simulink model "Energy_Cost"  (Simulink 8.8)
settings: Solver=ode23t  StartTime=0.0  StopTime=24  RelTol=1e-3  EnableMultiTasking=on
model workspace: external: MAT-File (data not in the file)
libraries: simulink x4
(part 2 of 5)

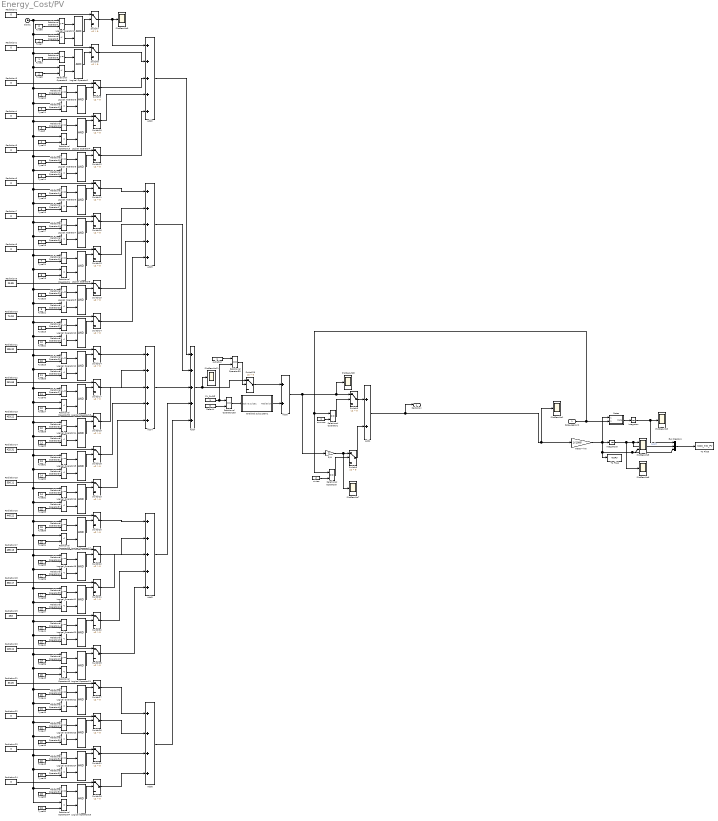
== system Energy_Cost/PV ==
  Rate_season2 : Inport
  Add1 : Sum
  Add{2..5,7} (5 alike) : Sum  Inputs=+++++
  Add6 : Sum  Inputs=++++
  Add8 : Sum
  Bus Creator4 : BusCreator  Inputs=3
  Clock1 : Clock
  Default : Constant  Value=0
  Enabled Subsystem1 : Subsystem  TreatAsAtomicUnit=on
  Integrator : Integrator
  Integrator3 : Integrator
  Logical Operator{1..18,20..25} (24 alike) : Logic  AllPortsSameDT=off  OutDataTypeStr=boolean
  PV_OnOff : Constant
  PlotResults{1,3,6..9,11} (7 alike) : Scope
  PlotResults5 : Scope  NumInputPorts=2
  Radiation{1..8,22..24} (11 alike) : Constant  Value=0
  Radiation10 : Constant  Value=74.18
  Radiation11 : Constant  Value=195.32
  Radiation12 : Constant  Value=281.63
  Radiation13 : Constant  Value=453.22
  Radiation14 : Constant  Value=425.31
  Radiation15 : Constant  Value=556.11
  Radiation16 : Constant  Value=445.22
  Radiation17 : Constant  Value=485.13
  Radiation18 : Constant  Value=360.17
  Radiation19 : Constant  Value=253
  Radiation20 : Constant  Value=126.11
  Radiation21 : Constant  Value=33.25
  Radiation9 : Constant  Value=25.85
  Rates : Subsystem
  Relational Operator{1,5,55,103} (4 alike) : RelationalOperator  Operator===  RndMeth=Nearest  InputSameDT=on
  Relational Operator{6..7,10..11,14..15,18..19,22..23,27..28,31..32,35..36,39..40,43..44,47..48,51..52} (24 alike) : RelationalOperator  RndMeth=Nearest  InputSameDT=on
  Relational Operator{8..9,12..13,16..17,20..21,25..26,29..30,33..34,37..38,41..42,45..46,49..50,53..54} (24 alike) : RelationalOperator  Operator=<  RndMeth=Nearest  InputSameDT=on
  S\W : Gain  Gain=.5  SaturateOnIntegerOverflow=on  OutDataTypeStr=Inherit: Same as input  ParamDataTypeStr=Inherit: Same as input
  Switch{5..29,31..32} (27 alike) : Switch  Criteria=u2 > Threshold
  To File1 : ToFile  Filename=TinPV  MatrixName=TinPV
  To File5 : ToFile  Filename=Cost_KW_PV  MatrixName=Cost_KW_PV
  Type10 : Constant  Value=2
  Type11 : Constant  Value=3
  Type12 : Constant  Value=4
  Type13 : Constant  Value=4
  Type14 : Constant  Value=5
  Type15 : Constant  Value=6
  Type16 : Constant  Value=5
  Type17 : Constant  Value=6
  Type18 : Constant  Value=7
  Type19 : Constant  Value=8
  Type2 : Constant
  Type20 : Constant  Value=8
  Type21 : Constant  Value=9
  Type22 : Constant  Value=10
  Type23 : Constant  Value=9
  Type24 : Constant  Value=7
  Type25 : Constant  Value=10
  Type26 : Constant  Value=11
  Type27 : Constant  Value=12
  Type28 : Constant  Value=12
  Type29 : Constant  Value=13
  Type30 : Constant  Value=14
  Type31 : Constant  Value=13
  Type32 : Constant  Value=14
  Type33 : Constant  Value=15
  Type34 : Constant  Value=16
  Type35 : Constant  Value=16
  Type36 : Constant  Value=17
  Type37 : Constant  Value=18
  Type38 : Constant  Value=17
  Type39 : Constant  Value=15
  Type40 : Constant  Value=11
  Type41 : Constant  Value=18
  Type42 : Constant  Value=19
  Type43 : Constant  Value=20
  Type44 : Constant  Value=20
  Type45 : Constant  Value=21
  Type46 : Constant  Value=22
  Type47 : Constant  Value=21
  Type48 : Constant  Value=22
  Type49 : Constant  Value=23
  Type50 : Constant  Value=24
  Type55 : Constant  Value=23
  Type56 : Constant  Value=19
  Type6 : Constant  Value=0
  Type7 : Constant
  Type8 : Constant  Value=2
  Type9 : Constant  Value=3
  Watts-->kW : Gain  Gain=1/(1000)  SaturateOnIntegerOverflow=on  OutDataTypeStr=Inherit: Same as input  ParamDataTypeStr=Inherit: Same as input
  radiation : Constant
  summer : Constant
  winter : Constant  Value=2
  Radiation : Outport
  wires:
  Add1/1 -> PlotResults1/1, Watts-->kW/1, Radiation/1
  Integrator3/1 -> PlotResults5/1, Bus Creator4/2, PlotResults6/1  "kw-hr"
  Watts-->kW/1 -> Integrator3/1, Rates/1(Powe_cons), To File1/1, Bus Creator4/3, PlotResults5/2
  Rates/1(Rate) -> Integrator/1
  Integrator/1 -> PlotResults3/1, Bus Creator4/1
  Rate_season2/1 -> Rates/2(Rate_season2), Relational Operator1/1, Relational Operator5/1
  Relational Operator1/1 -> Switch5/2
  summer/1 -> Relational Operator1/2
  Switch5/1 -> Add1/1
  Relational Operator5/1 -> Switch6/2
  winter/1 -> Relational Operator5/2
  Switch6/1 -> Add1/2
  S\W/1 -> Switch6/1, PlotResults7/1
  Bus Creator4/1 -> To File5/1
  Radiation1/1 -> Switch7/1
  Switch7/1 -> PlotResults9/1, Add2/1
  Clock1/1 -> Relational Operator7/1, Relational Operator8/1, Relational Operator6/1, Relational Operator9/1, Relational Operator19/1, Relational Operator20/1, Relational Operator18/1, Relational Operator21/1, Relational Operator23/1, Relational Operator25/1, Relational Operator22/1, Relational Operator26/1, Relational Operator28/1, Relational Operator29/1, Relational Operator27/1, Relational Operator32/1, Relational Operator31/1, Relational Operator34/1, Relational Operator36/1, Relational Operator37/1, Relational Operator35/1, Relational Operator38/1, Relational Operator40/1, Relational Operator41/1, Relational Operator39/1, Relational Operator42/1, Relational Operator45/1, Relational Operator43/1, Relational Operator47/1, Relational Operator54/1, Relational Operator51/1, Relational Operator53/1, Relational Operator52/1, Relational Operator50/1, Relational Operator49/1, Relational Operator48/1, Relational Operator46/1, Relational Operator44/1, Relational Operator33/1, Relational Operator30/1, Relational Operator17/1, Relational Operator14/1, Relational Operator16/1, Relational Operator15/1, Relational Operator13/1, Relational Operator10/1, Relational Operator12/1, Relational Operator11/1
  Type6/1 -> Relational Operator7/2
  Type7/1 -> Relational Operator8/2
  Relational Operator8/1 -> Logical Operator1/2
  Relational Operator7/1 -> Logical Operator1/1
  Logical Operator1/1 -> Switch7/2
  Radiation2/1 -> Switch8/1
  Type2/1 -> Relational Operator6/2
  Type8/1 -> Relational Operator9/2
  Relational Operator9/1 -> Logical Operator2/2
  Relational Operator6/1 -> Logical Operator2/1
  Logical Operator2/1 -> Switch8/2
  Type10/1 -> Relational Operator11/2
  Type11/1 -> Relational Operator12/2
  Relational Operator12/1 -> Logical Operator3/2
  Relational Operator11/1 -> Logical Operator3/1
  Logical Operator3/1 -> Switch9/2
  Type9/1 -> Relational Operator10/2
  Type12/1 -> Relational Operator13/2
  Relational Operator13/1 -> Logical Operator4/2
  Relational Operator10/1 -> Logical Operator4/1
  Logical Operator4/1 -> Switch10/2
  Type13/1 -> Relational Operator15/2
  Type14/1 -> Relational Operator16/2
  Relational Operator16/1 -> Logical Operator5/2
  Relational Operator15/1 -> Logical Operator5/1
  Logical Operator5/1 -> Switch12/2
  Type16/1 -> Relational Operator14/2
  Type15/1 -> Relational Operator17/2
  Relational Operator17/1 -> Logical Operator6/2
  Relational Operator14/1 -> Logical Operator6/1
  Logical Operator6/1 -> Switch11/2
  Type17/1 -> Relational Operator19/2
  Type18/1 -> Relational Operator20/2
  Relational Operator20/1 -> Logical Operator7/2
  Relational Operator19/1 -> Logical Operator7/1
  Logical Operator7/1 -> Switch16/2
  Type24/1 -> Relational Operator18/2
  Type19/1 -> Relational Operator21/2
  Relational Operator21/1 -> Logical Operator8/2
  Relational Operator18/1 -> Logical Operator8/1
  Logical Operator8/1 -> Switch13/2
  Type20/1 -> Relational Operator23/2
  Type21/1 -> Relational Operator25/2
  Relational Operator25/1 -> Logical Operator9/2
  Relational Operator23/1 -> Logical Operator9/1
  Logical Operator9/1 -> Switch15/2
  Type23/1 -> Relational Operator22/2
  Type22/1 -> Relational Operator26/2
  Relational Operator26/1 -> Logical Operator10/2
  Relational Operator22/1 -> Logical Operator10/1
  Logical Operator10/1 -> Switch14/2
  Type25/1 -> Relational Operator28/2
  Type26/1 -> Relational Operator29/2
  Relational Operator29/1 -> Logical Operator12/2
  Relational Operator28/1 -> Logical Operator12/1
  Logical Operator12/1 -> Switch24/2
  Type40/1 -> Relational Operator27/2
  Type27/1 -> Relational Operator30/2
  Relational Operator30/1 -> Logical Operator13/2
  Relational Operator27/1 -> Logical Operator13/1
  Logical Operator13/1 -> Switch17/2
  Type28/1 -> Relational Operator32/2
  Type29/1 -> Relational Operator33/2
  Relational Operator33/1 -> Logical Operator14/2
  Relational Operator32/1 -> Logical Operator14/1
  Logical Operator14/1 -> Switch19/2
  Type31/1 -> Relational Operator31/2
  Type30/1 -> Relational Operator34/2
  Relational Operator34/1 -> Logical Operator15/2
  Relational Operator31/1 -> Logical Operator15/1
  Logical Operator15/1 -> Switch18/2
  Type32/1 -> Relational Operator36/2
  Type33/1 -> Relational Operator37/2
  Relational Operator37/1 -> Logical Operator16/2
  Relational Operator36/1 -> Logical Operator16/1
  Logical Operator16/1 -> Switch23/2
  Type39/1 -> Relational Operator35/2
  Type34/1 -> Relational Operator38/2
  Relational Operator38/1 -> Logical Operator17/2
  Relational Operator35/1 -> Logical Operator17/1
  Logical Operator17/1 -> Switch20/2
  Type35/1 -> Relational Operator40/2
  Type36/1 -> Relational Operator41/2
  Relational Operator41/1 -> Logical Operator18/2
  Relational Operator40/1 -> Logical Operator18/1
  Logical Operator18/1 -> Switch22/2
  Type38/1 -> Relational Operator39/2
  Type37/1 -> Relational Operator42/2
  Relational Operator42/1 -> Logical Operator11/2
  Relational Operator39/1 -> Logical Operator11/1
  Logical Operator11/1 -> Switch21/2
  Type41/1 -> Relational Operator44/2
  Type42/1 -> Relational Operator45/2
  Relational Operator45/1 -> Logical Operator20/2
  Relational Operator44/1 -> Logical Operator20/1
  Logical Operator20/1 -> Switch32/2
  Type56/1 -> Relational Operator43/2
  Type43/1 -> Relational Operator46/2
  Relational Operator46/1 -> Logical Operator21/2
  Relational Operator43/1 -> Logical Operator21/1
  Logical Operator21/1 -> Switch25/2
  Type44/1 -> Relational Operator48/2
  Type45/1 -> Relational Operator49/2
  Relational Operator49/1 -> Logical Operator22/2
  Relational Operator48/1 -> Logical Operator22/1
  Logical Operator22/1 -> Switch27/2
  Type47/1 -> Relational Operator47/2
  Type46/1 -> Relational Operator50/2
  Relational Operator50/1 -> Logical Operator23/2
  Relational Operator47/1 -> Logical Operator23/1
  Logical Operator23/1 -> Switch26/2
  Type48/1 -> Relational Operator52/2
  Type49/1 -> Relational Operator53/2
  Relational Operator53/1 -> Logical Operator24/2
  Relational Operator52/1 -> Logical Operator24/1
  Logical Operator24/1 -> Switch31/2
  Type55/1 -> Relational Operator51/2
  Type50/1 -> Relational Operator54/2
  Relational Operator54/1 -> Logical Operator25/2
  Relational Operator51/1 -> Logical Operator25/1
  Logical Operator25/1 -> Switch28/2
  Radiation3/1 -> Switch9/1
  Radiation4/1 -> Switch10/1
  Radiation5/1 -> Switch12/1
  Radiation6/1 -> Switch11/1
  Radiation7/1 -> Switch16/1
  Radiation8/1 -> Switch13/1
  Radiation9/1 -> Switch15/1
  Radiation10/1 -> Switch14/1
  Radiation11/1 -> Switch24/1
  Radiation12/1 -> Switch17/1
  Radiation13/1 -> Switch19/1
  Radiation14/1 -> Switch18/1
  Radiation15/1 -> Switch23/1
  Radiation16/1 -> Switch20/1
  Radiation17/1 -> Switch22/1
  Radiation18/1 -> Switch21/1
  Radiation19/1 -> Switch32/1
  Radiation20/1 -> Switch25/1
  Radiation21/1 -> Switch27/1
  Radiation22/1 -> Switch26/1
  Radiation23/1 -> Switch31/1
  Radiation24/1 -> Switch28/1
  Switch8/1 -> Add2/2
  Switch9/1 -> Add2/3
  Switch12/1 -> Add2/5
  Switch10/1 -> Add2/4
  Switch11/1 -> Add3/1
  Switch16/1 -> Add3/2
  Switch13/1 -> Add3/3
  Switch15/1 -> Add3/4
  Switch14/1 -> Add3/5
  Switch24/1 -> Add4/1
  Switch17/1 -> Add4/2
  Switch19/1 -> Add4/3
  Switch18/1 -> Add4/4
  Switch23/1 -> Add4/5
  Switch20/1 -> Add5/1
  Switch22/1 -> Add5/2
  Switch21/1 -> Add5/3
  Switch32/1 -> Add5/4
  Switch25/1 -> Add5/5
  Switch27/1 -> Add6/1
  Switch26/1 -> Add6/2
  Switch31/1 -> Add6/3
  Switch28/1 -> Add6/4
  Add2/1 -> Add7/1
  Add3/1 -> Add7/2
  Add4/1 -> Add7/3
  Add5/1 -> Add7/4
  Add6/1 -> Add7/5
  Add8/1 -> Switch5/1, PlotResults8/1, S\W/1
  Default/1 -> Relational Operator103/2
  Relational Operator103/1 -> Enabled Subsystem1/1(active pulse1)
  PV_OnOff/1 -> Relational Operator103/1, Relational Operator55/2
  Enabled Subsystem1/1(Radiation) -> Add8/2
  Relational Operator55/1 -> Switch29/2
  radiation/1 -> Relational Operator55/1
  Add7/1 -> Switch29/1, PlotResults11/1
  Switch29/1 -> Add8/1

== system Energy_Cost/PoolPump ==
  Bus Creator : BusCreator  Inputs=6
  LoadsDay : Constant  Value=3
  MinOfLoad : Constant  Value=180
  PP_OnOff : Constant
  Terminator : Terminator
  WhenUsed1 : Constant  Value=5
  WhenUsed2 : Constant  Value=14
  WhenUsed3 : Constant  Value=22
  wires:
  PP_OnOff/1 -> Bus Creator/1
  Bus Creator/1 -> Terminator/1
  WhenUsed3/1 -> Bus Creator/6
  WhenUsed2/1 -> Bus Creator/5
  WhenUsed1/1 -> Bus Creator/4
  MinOfLoad/1 -> Bus Creator/3
  LoadsDay/1 -> Bus Creator/2

== system Energy_Cost/Range ==
  B1 : Constant  Value=0.6
  B2 : Constant  Value=0.4
  B3 : Constant  Value=0.4
  B4 : Constant  Value=0.6
  Bus Creator1 : BusCreator  Inputs=9
  Bus Creator2 : BusCreator  Inputs=6
  OnOff_Range : Constant
  SB{1..4} (4 alike) : Constant  Value=1200
  TOU_Mor1 : Constant  Value=0.66667
  TOU_Nig1 : Constant  Value=0.5
  TOU_Noon1 : Constant  Value=1.5
  Terminator1 : Terminator
  Terminator2 : Terminator
  switchedOn_Mor1 : Constant  Value=7
  switchedOn_Nig1 : Constant  Value=20.3
  switchedOn_Noon1 : Constant  Value=14
  wires:
  B1/1 -> Bus Creator1/1
  SB1/1 -> Bus Creator1/2
  B2/1 -> Bus Creator1/3
  SB2/1 -> Bus Creator1/4
  B3/1 -> Bus Creator1/5
  SB3/1 -> Bus Creator1/6
  B4/1 -> Bus Creator1/7
  SB4/1 -> Bus Creator1/8
  TOU_Mor1/1 -> Bus Creator2/1
  switchedOn_Mor1/1 -> Bus Creator2/2
  TOU_Noon1/1 -> Bus Creator2/3
  switchedOn_Noon1/1 -> Bus Creator2/4
  TOU_Nig1/1 -> Bus Creator2/5
  switchedOn_Nig1/1 -> Bus Creator2/6
  Bus Creator2/1 -> Terminator2/1
  Bus Creator1/1 -> Terminator1/1
  OnOff_Range/1 -> Bus Creator1/9

== system Energy_Cost/Ref Therm ==
  Tamb : Inport
  Tamb1 : Inport  Port=2
  Sum3 : Sum  Inputs=|+-  SaturateOnIntegerOverflow=on  InputSameDT=on  OutDataTypeStr=Inherit: Same as first input
  Thermostat1 : Relay  OnSwitchValue=1.5  OffSwitchValue=-1.5  OnOutputValue=0  OffOutputValue=1  ZeroCross=off
  Ref Therm : Outport  InitialOutput=0
  wires:
  Sum3/1 -> Thermostat1/1
  Thermostat1/1 -> Ref Therm/1
  Tamb/1 -> Sum3/1
  Tamb1/1 -> Sum3/2

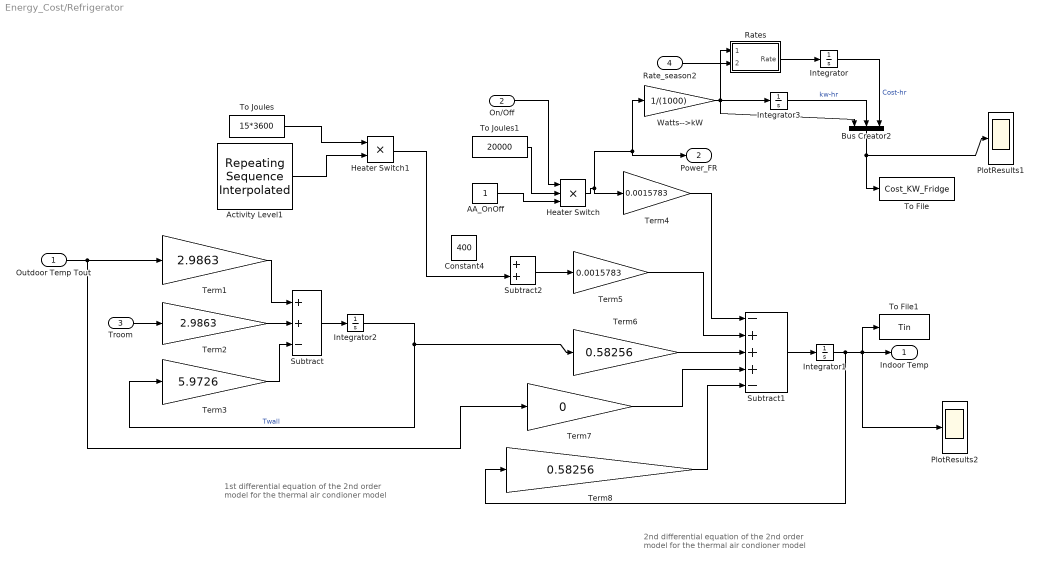
== system Energy_Cost/Refrigerator ==
  note: 1st differential equation of the 2nd order
      | model for the thermal air condioner model
  note: 2nd differential equation of the 2nd order
      | model for the thermal air condioner model
  Outdoor Temp Tout : Inport
  On/Off : Inport  Port=2
  Troom : Inport  Port=3
  Rate_season2 : Inport  Port=4
  AA_OnOff : Constant
  Activity Level1 : simulink/Sources/Repeating Sequence Interpolated  OutValues=|  TimeValues=|  LookUpMeth=Interpolation-Use End Values  tsamp=1  OutMin=[]  OutMax=[]  OutDataTypeStr=double  OutputDataTypeScalingMode=double  OutDataType=fixdt(0,8)  OutScaling=2^-10
      OutValues=|
      | [         0
      |          0
      |     0.0700
      |     0.0700
      |          0
      |          0
      |     0.1000
      |     0.1000
      |          0
      |          0
      |     0.1300
      |     0.1300
      |          0
      |          0
      |     0.0300
      |     0.0300
      |          0
      |          0
      |          0
      |     0.0700
      |     0.0700
      |          0
      |          0
      |     0.1700
      |     0.1700
      |          0
      |          0
      |     0.2300
      |     0.2300
      |          0
      |          0
      |     0.1300
      |     0.1300
      |          0
      |          0
      |     0.0700
      |     0.0700
      |          0
      |          0].'
      TimeValues=|
      | [                   0
      |    9.299899999999999
      |    9.300000000000001
      |    9.303990000000001
      |    9.304000000000000
      |    9.749000000000001
      |    9.750000000000000
      |    9.755000000000001
      |    9.756000000000000
      |    9.999000000000001
      |   10.000000000000000
      |   10.006700000000000
      |   10.006800000000000
      |   10.149900000000001
      |   10.150000000000000
      |   10.151600000000000
      |   10.151700000000000
      |   10.300100000000000
      |   13.299899999999999
      |   13.300000000000001
      |   13.303300000000000
      |   13.303400000000000
      |   13.449900000000000
      |   13.449999999999999
      |   13.458399999999999
      |   13.458500000000001
      |   13.999900000000000
      |   14.000000000000000
      |   14.011690000000000
      |   14.011699999999999
      |   14.149900000000001
      |   14.150000000000000
      |   14.156700000000001
      |   14.156800000000000
      |   14.299899999999999
      |   14.300000000000001
      |   14.303300000000000
      |   14.303400000000000
      |   24.000000000000000].'
  Bus Creator2 : BusCreator  Inputs=3
  Constant4 : Constant  Value=400
  Heater Switch : Product  Inputs=3  RndMeth=Zero
  Heater Switch1 : Product  RndMeth=Zero
  Integrator : Integrator
  Integrator1 : Integrator  InitialCondition=4
  Integrator2 : Integrator  InitialCondition=21
  Integrator3 : Integrator
  PlotResults1 : Scope
  PlotResults2 : Scope
  Rates : Subsystem
  Subtract : Sum  Inputs=++-
  Subtract1 : Sum  Inputs=-+++-
  Subtract2 : Sum
  Term1 : Gain  Gain=2.9863
  Term2 : Gain  Gain=2.9863
  Term3 : Gain  Gain=5.9726
  Term4 : Gain  Gain=0.0015783
  Term5 : Gain  Gain=0.0015783
  Term6 : Gain  Gain=0.58256
  Term7 : Gain  Gain=0
  Term8 : Gain  Gain=0.58256
  To File : ToFile  Filename=Cost_KW_Fridge  MatrixName=Cost_KW_Fridge
  To File1 : ToFile  Filename=Tin  MatrixName=Tin
  To Joules : Constant  Value=15*3600
  To Joules1 : Constant  Value=20000
  Watts-->kW : Gain  Gain=1/(1000)  SaturateOnIntegerOverflow=on  OutDataTypeStr=Inherit: Same as input  ParamDataTypeStr=Inherit: Same as input
  Indoor Temp : Outport  InitialOutput=0
  Power_FR : Outport  Port=2  InitialOutput=0
  wires:
  Term3/1 -> Subtract/3
  Subtract/1 -> Integrator2/1
  Integrator2/1 -> Term3/1, Term6/1  "Twall"
  Integrator1/1 -> Indoor Temp/1, To File1/1, PlotResults2/1, Term8/1
  Subtract1/1 -> Integrator1/1
  Outdoor Temp Tout/1 -> Term7/1, Term1/1
  Troom/1 -> Term2/1
  Term5/1 -> Subtract1/2
  Term6/1 -> Subtract1/3
  Term7/1 -> Subtract1/4
  Term8/1 -> Subtract1/5
  To Joules/1 -> Heater Switch1/1
  Heater Switch1/1 -> Subtract2/2
  On/Off/1 -> Heater Switch/1
  Subtract2/1 -> Term5/1
  Term1/1 -> Subtract/1
  Term2/1 -> Subtract/2
  To Joules1/1 -> Heater Switch/2
  Heater Switch/1 -> Term4/1, Power_FR/1, Watts-->kW/1
  Term4/1 -> Subtract1/1
  Rates/1(Rate) -> Integrator/1
  Watts-->kW/1 -> Integrator3/1, Rates/1(Powe_cons), Bus Creator2/1
  Integrator3/1 -> Bus Creator2/2  "kw-hr"
  Bus Creator2/1 -> To File/1, PlotResults1/1
  Integrator/1 -> Bus Creator2/3  "Cost-hr"
  AA_OnOff/1 -> Heater Switch/3
  Activity Level1/1 -> Heater Switch1/2
  Rate_season2/1 -> Rates/2(Rate_season2)

== system Energy_Cost/Thermostat ==
  Clock3 : Clock
      settings: Decimation=100
  If : If  IfExpression=u1 == 0
  If Action Subsystem : Subsystem  TreatAsAtomicUnit=on
  If Action Subsystem1 : Subsystem  TreatAsAtomicUnit=on
  Merge : Merge
  P1_on : Constant  Value=8
  P1_set : Constant  Value=23
  P2_on : Constant  Value=15
  P2_set : Constant  Value=23
  P3_on : Constant  Value=21
  P3_set : Constant  Value=23
  P4_on : Constant  Value=16
  P4_set : Constant  Value=23
  Sche : Constant
  Set_Point_AA : Constant  Value=2.5
  Temperatures2 : Scope
  Thermostat_Schedule : M-S-Function  FunctionName=Thermostat_Schedule
  To File : ToFile  Filename=Term_Smart  MatrixName=Term_Smart
  Sche_SetP : Outport  InitialOutput=0
  wires:
  P1_on/1 -> Thermostat_Schedule/1
  P1_set/1 -> Thermostat_Schedule/2
  P2_on/1 -> Thermostat_Schedule/3
  P2_set/1 -> Thermostat_Schedule/4
  P3_on/1 -> Thermostat_Schedule/5
  P3_set/1 -> Thermostat_Schedule/6
  P4_on/1 -> Thermostat_Schedule/7
  P4_set/1 -> Thermostat_Schedule/8
  Clock3/1 -> Thermostat_Schedule/9
  Sche/1 -> If/1
  If/1 -> If Action Subsystem/Action
  Set_Point_AA/1 -> If Action Subsystem/1(In1)
  If/2 -> If Action Subsystem1/Action
  Merge/1 -> Sche_SetP/1, Temperatures2/1, To File/1
  Thermostat_Schedule/1 -> If Action Subsystem1/1(In1)
  If Action Subsystem1/1(Out1) -> Merge/2
  If Action Subsystem/1(Out1) -> Merge/1

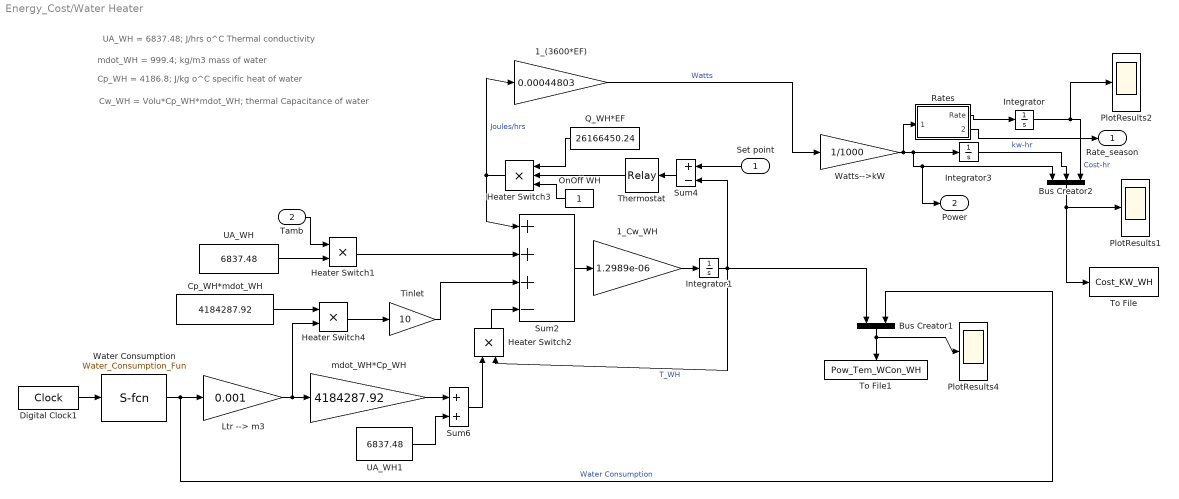
== system Energy_Cost/Water Heater ==
  note: UA_WH = 6837.48; J/hrs o^C Thermal conductivity
  note: mdot_WH = 999.4; kg/m3 mass of water
  note: Cp_WH = 4186.8; J/kg o^C specific heat of water
  note: Cw_WH = Volu*Cp_WH*mdot_WH; thermal Capacitance of water
  Set point : Inport
  Tamb : Inport  Port=2
  1_(3600*EF) : Gain  Gain=0.00044803  SaturateOnIntegerOverflow=on  OutDataTypeStr=Inherit: Same as input  ParamDataTypeStr=Inherit: Same as input
  1_Cw_WH : Gain  Gain=1.2989e-06  SaturateOnIntegerOverflow=on  OutDataTypeStr=Inherit: Same as input  ParamDataTypeStr=Inherit: Same as input
  Bus Creator1 : BusCreator  Inputs=2
  Bus Creator2 : BusCreator  Inputs=3
  Cp_WH*mdot_WH : Constant  Value=4184287.92
  Digital Clock1 : DigitalClock
  Heater Switch1 : Product  RndMeth=Zero
  Heater Switch2 : Product  RndMeth=Zero
  Heater Switch3 : Product  Inputs=3  RndMeth=Zero
  Heater Switch4 : Product  RndMeth=Zero
  Integrator : Integrator
  Integrator1 : Integrator  InitialCondition=55
  Integrator3 : Integrator
  Ltr --> m3 : Gain  Gain=0.001
  OnOff WH : Constant  VectorParams1D=off
  PlotResults1 : Scope
  PlotResults2 : Scope
  PlotResults4 : Scope
  Q_WH*EF : Constant  Value=26166450.24  VectorParams1D=off
  Rates : Subsystem
  Sum2 : Sum  Inputs=+++-  SaturateOnIntegerOverflow=on  InputSameDT=on  OutDataTypeStr=Inherit: Same as first input
  Sum4 : Sum  Inputs=+-  SaturateOnIntegerOverflow=on  InputSameDT=on  OutDataTypeStr=Inherit: Same as first input
  Sum6 : Sum  SaturateOnIntegerOverflow=on  InputSameDT=on  OutDataTypeStr=Inherit: Same as first input
  Thermostat : Relay  OnSwitchValue=3  OffSwitchValue=-3
  Tinlet : Gain  Gain=10  SaturateOnIntegerOverflow=on  OutDataTypeStr=Inherit: Same as input  ParamDataTypeStr=Inherit: Same as input
  To File : ToFile  Filename=Cost_KW_WH  MatrixName=Cost_KW_WH
  To File1 : ToFile  Filename=Pow_Tem_WCon_WH  MatrixName=Pow_Tem_WCon_WH
  UA_WH : Constant  Value=6837.48
  UA_WH1 : Constant  Value=6837.48
  Water Consumption : M-S-Function  FunctionName=Water_Consumption_Fun
  Watts-->kW : Gain  Gain=1/1000  SaturateOnIntegerOverflow=on  OutDataTypeStr=Inherit: Same as input  ParamDataTypeStr=Inherit: Same as input
  mdot_WH*Cp_WH : Gain  Gain=4184287.92  SaturateOnIntegerOverflow=on  OutDataTypeStr=Inherit: Same as input  ParamDataTypeStr=Inherit: Same as input
  Rate_season : Outport  InitialOutput=0
  Power : Outport  Port=2  InitialOutput=0
  wires:
  Sum2/1 -> 1_Cw_WH/1
  1_Cw_WH/1 -> Integrator1/1
  Digital Clock1/1 -> Water Consumption/1
  Water Consumption/1 -> Ltr --> m3/1, Bus Creator1/2  "Water Consumption"
  UA_WH/1 -> Heater Switch1/2
  Ltr --> m3/1 -> mdot_WH*Cp_WH/1, Heater Switch4/2
  mdot_WH*Cp_WH/1 -> Sum6/1
  UA_WH1/1 -> Sum6/2
  Sum6/1 -> Heater Switch2/1
  Integrator1/1 -> Heater Switch2/2, Sum4/2, Bus Creator1/1  "T_WH"
  Heater Switch2/1 -> Sum2/4
  Cp_WH*mdot_WH/1 -> Heater Switch4/1
  Heater Switch4/1 -> Tinlet/1
  Tinlet/1 -> Sum2/3
  Heater Switch1/1 -> Sum2/2
  Set point/1 -> Sum4/1
  Sum4/1 -> Thermostat/1
  Q_WH*EF/1 -> Heater Switch3/1
  Heater Switch3/1 -> Sum2/1, 1_(3600*EF)/1  "Joules/hrs"
  1_(3600*EF)/1 -> Watts-->kW/1  "Watts"
  Thermostat/1 -> Heater Switch3/2
  Tamb/1 -> Heater Switch1/1
  Rates/1(Rate) -> Integrator/1
  Watts-->kW/1 -> Rates/1(Powe_cons), Integrator3/1, Bus Creator2/1, Power/1
  Integrator3/1 -> Bus Creator2/2  "kw-hr"
  Bus Creator2/1 -> To File/1, PlotResults1/1
  Bus Creator1/1 -> To File1/1, PlotResults4/1
  Integrator/1 -> PlotResults2/1, Bus Creator2/3  "Cost-hr"
  OnOff WH/1 -> Heater Switch3/3
  Rates/2(Rate_season1) -> Rate_season/1

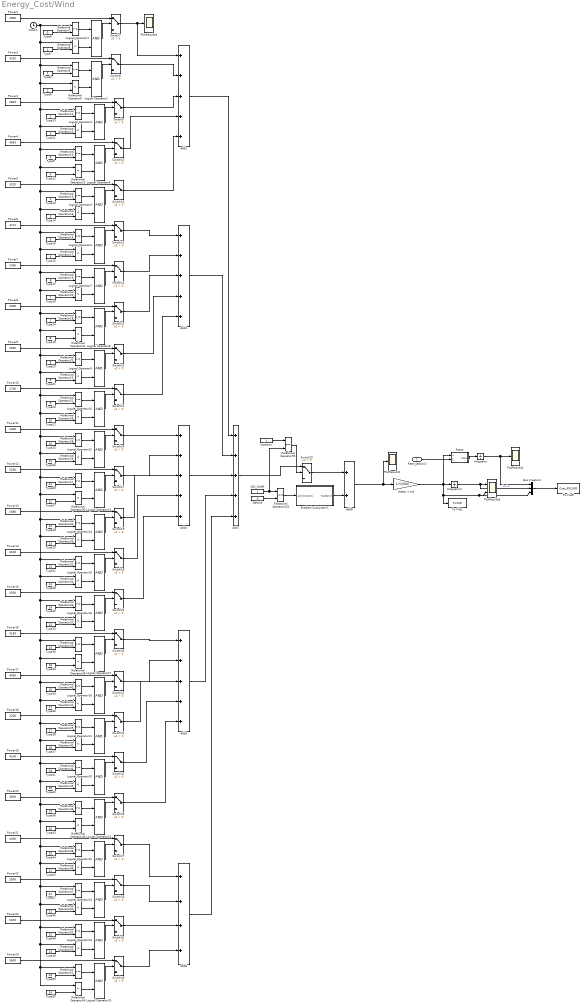
== system Energy_Cost/Wind ==
  Rate_season2 : Inport
  Add{2..5,7} (5 alike) : Sum  Inputs=+++++
  Add6 : Sum  Inputs=++++
  Add8 : Sum
  Bus Creator4 : BusCreator  Inputs=3
  Clock1 : Clock
  Default : Constant  Value=0
  Enabled Subsystem1 : Subsystem  TreatAsAtomicUnit=on
  Integrator : Integrator
  Integrator3 : Integrator
  Logical Operator{1..18,20..25} (24 alike) : Logic  AllPortsSameDT=off  OutDataTypeStr=boolean
  PlotResults2 : Scope
  PlotResults3 : Scope
  PlotResults5 : Scope  NumInputPorts=2
  PlotResults9 : Scope
  Power1 : Constant  Value=2965
  Power10 : Constant  Value=1700
  Power11 : Constant  Value=2440
  Power12 : Constant  Value=2250
  Power13 : Constant  Value=2680
  Power14 : Constant  Value=3100
  Power15 : Constant  Value=4500
  Power16 : Constant  Value=5150
  Power17 : Constant  Value=4550
  Power18 : Constant  Value=3200
  Power19 : Constant  Value=4100
  Power2 : Constant  Value=4220
  Power20 : Constant  Value=3600
  Power21 : Constant  Value=4000
  Power22 : Constant  Value=2600
  Power23 : Constant  Value=5220
  Power24 : Constant  Value=3600
  Power3 : Constant  Value=2825
  Power4 : Constant  Value=4555
  Power5 : Constant  Value=3220
  Power6 : Constant  Value=3711
  Power7 : Constant  Value=2430
  Power8 : Constant  Value=2000
  Power9 : Constant  Value=2650
  Rates : Subsystem
  Relational Operator{6..7,10..11,14..15,18..19,22..23,27..28,31..32,35..36,39..40,43..44,47..48,51..52} (24 alike) : RelationalOperator  RndMeth=Nearest  InputSameDT=on
  Relational Operator103 : RelationalOperator  Operator===  RndMeth=Nearest  InputSameDT=on
  Relational Operator{8..9,12..13,16..17,20..21,25..26,29..30,33..34,37..38,41..42,45..46,49..50,53..54} (24 alike) : RelationalOperator  Operator=<  RndMeth=Nearest  InputSameDT=on
  Relational Operator55 : RelationalOperator  Operator===  RndMeth=Nearest  InputSameDT=on
  Switch{7..29,31..32} (25 alike) : Switch  Criteria=u2 > Threshold
  To File1 : ToFile  Filename=TinWD  MatrixName=TinWD
  To File5 : ToFile  Filename=Cost_KW_WD  MatrixName=Cost_KW_WD
  Type10 : Constant  Value=2
  Type11 : Constant  Value=3
  Type12 : Constant  Value=4
  Type13 : Constant  Value=4
  Type14 : Constant  Value=5
  Type15 : Constant  Value=6
  Type16 : Constant  Value=5
  Type17 : Constant  Value=6
  Type18 : Constant  Value=7
  Type19 : Constant  Value=8
  Type2 : Constant
  Type20 : Constant  Value=8
  Type21 : Constant  Value=9
  Type22 : Constant  Value=10
  Type23 : Constant  Value=9
  Type24 : Constant  Value=7
  Type25 : Constant  Value=10
  Type26 : Constant  Value=11
  Type27 : Constant  Value=12
  Type28 : Constant  Value=12
  Type29 : Constant  Value=13
  Type30 : Constant  Value=14
  Type31 : Constant  Value=13
  Type32 : Constant  Value=14
  Type33 : Constant  Value=15
  Type34 : Constant  Value=16
  Type35 : Constant  Value=16
  Type36 : Constant  Value=17
  Type37 : Constant  Value=18
  Type38 : Constant  Value=17
  Type39 : Constant  Value=15
  Type40 : Constant  Value=11
  Type41 : Constant  Value=18
  Type42 : Constant  Value=19
  Type43 : Constant  Value=20
  Type44 : Constant  Value=20
  Type45 : Constant  Value=21
  Type46 : Constant  Value=22
  Type47 : Constant  Value=21
  Type48 : Constant  Value=22
  Type49 : Constant  Value=23
  Type50 : Constant  Value=24
  Type55 : Constant  Value=23
  Type56 : Constant  Value=19
  Type6 : Constant  Value=0
  Type7 : Constant
  Type8 : Constant  Value=2
  Type9 : Constant  Value=3
  WD_OnOff : Constant
  Watts-->kW : Gain  Gain=1/(1000)  SaturateOnIntegerOverflow=on  OutDataTypeStr=Inherit: Same as input  ParamDataTypeStr=Inherit: Same as input
  radiation : Constant
  wires:
  Type36/1 -> Relational Operator41/2
  Relational Operator41/1 -> Logical Operator18/2
  Type38/1 -> Relational Operator39/2
  Type37/1 -> Relational Operator42/2
  Relational Operator42/1 -> Logical Operator11/2
  Relational Operator39/1 -> Logical Operator11/1
  Logical Operator11/1 -> Switch21/2
  Type41/1 -> Relational Operator44/2
  Type42/1 -> Relational Operator45/2
  Relational Operator45/1 -> Logical Operator20/2
  Relational Operator44/1 -> Logical Operator20/1
  Logical Operator20/1 -> Switch32/2
  Type56/1 -> Relational Operator43/2
  Type43/1 -> Relational Operator46/2
  Relational Operator46/1 -> Logical Operator21/2
  Relational Operator43/1 -> Logical Operator21/1
  Logical Operator21/1 -> Switch25/2
  Type44/1 -> Relational Operator48/2
  Type45/1 -> Relational Operator49/2
  Relational Operator49/1 -> Logical Operator22/2
  Relational Operator48/1 -> Logical Operator22/1
  Logical Operator22/1 -> Switch27/2
  Type47/1 -> Relational Operator47/2
  Type46/1 -> Relational Operator50/2
  Relational Operator50/1 -> Logical Operator23/2
  Relational Operator47/1 -> Logical Operator23/1
  Logical Operator23/1 -> Switch26/2
  Type48/1 -> Relational Operator52/2
  Type49/1 -> Relational Operator53/2
  Relational Operator53/1 -> Logical Operator24/2
  Relational Operator52/1 -> Logical Operator24/1
  Logical Operator24/1 -> Switch31/2
  Type55/1 -> Relational Operator51/2
  Type50/1 -> Relational Operator54/2
  Relational Operator54/1 -> Logical Operator25/2
  Relational Operator51/1 -> Logical Operator25/1
  Logical Operator25/1 -> Switch28/2
  Power18/1 -> Switch21/1
  Power19/1 -> Switch32/1
  Power20/1 -> Switch25/1
  Power21/1 -> Switch27/1
  Power22/1 -> Switch26/1
  Power23/1 -> Switch31/1
  Power24/1 -> Switch28/1
  Switch32/1 -> Add5/4
  Switch25/1 -> Add5/5
  Switch27/1 -> Add6/1
  Switch26/1 -> Add6/2
  Switch31/1 -> Add6/3
  Switch28/1 -> Add6/4
  Power1/1 -> Switch7/1
  Switch7/1 -> PlotResults9/1, Add2/1
  Clock1/1 -> Relational Operator7/1, Relational Operator8/1, Relational Operator6/1, Relational Operator9/1, Relational Operator19/1, Relational Operator20/1, Relational Operator18/1, Relational Operator21/1, Relational Operator23/1, Relational Operator25/1, Relational Operator22/1, Relational Operator26/1, Relational Operator28/1, Relational Operator29/1, Relational Operator27/1, Relational Operator32/1, Relational Operator31/1, Relational Operator34/1, Relational Operator36/1, Relational Operator37/1, Relational Operator35/1, Relational Operator38/1, Relational Operator40/1, Relational Operator41/1, Relational Operator39/1, Relational Operator42/1, Relational Operator45/1, Relational Operator43/1, Relational Operator47/1, Relational Operator54/1, Relational Operator51/1, Relational Operator53/1, Relational Operator52/1, Relational Operator50/1, Relational Operator49/1, Relational Operator48/1, Relational Operator46/1, Relational Operator44/1, Relational Operator33/1, Relational Operator30/1, Relational Operator17/1, Relational Operator14/1, Relational Operator16/1, Relational Operator15/1, Relational Operator13/1, Relational Operator10/1, Relational Operator12/1, Relational Operator11/1
  Type6/1 -> Relational Operator7/2
  Type7/1 -> Relational Operator8/2
  Relational Operator8/1 -> Logical Operator1/2
  Relational Operator7/1 -> Logical Operator1/1
  Logical Operator1/1 -> Switch7/2
  Power2/1 -> Switch8/1
  Type2/1 -> Relational Operator6/2
  Type8/1 -> Relational Operator9/2
  Relational Operator9/1 -> Logical Operator2/2
  Relational Operator6/1 -> Logical Operator2/1
  Logical Operator2/1 -> Switch8/2
  Type10/1 -> Relational Operator11/2
  Type11/1 -> Relational Operator12/2
  Relational Operator12/1 -> Logical Operator3/2
  Relational Operator11/1 -> Logical Operator3/1
  Logical Operator3/1 -> Switch9/2
  Type9/1 -> Relational Operator10/2
  Type12/1 -> Relational Operator13/2
  Relational Operator13/1 -> Logical Operator4/2
  Relational Operator10/1 -> Logical Operator4/1
  Logical Operator4/1 -> Switch10/2
  Type13/1 -> Relational Operator15/2
  Type14/1 -> Relational Operator16/2
  Relational Operator16/1 -> Logical Operator5/2
  Relational Operator15/1 -> Logical Operator5/1
  Logical Operator5/1 -> Switch12/2
  Type16/1 -> Relational Operator14/2
  Type15/1 -> Relational Operator17/2
  Relational Operator17/1 -> Logical Operator6/2
  Relational Operator14/1 -> Logical Operator6/1
  Logical Operator6/1 -> Switch11/2
  Type17/1 -> Relational Operator19/2
  Type18/1 -> Relational Operator20/2
  Relational Operator20/1 -> Logical Operator7/2
  Relational Operator19/1 -> Logical Operator7/1
  Logical Operator7/1 -> Switch16/2
  Type24/1 -> Relational Operator18/2
  Type19/1 -> Relational Operator21/2
  Relational Operator21/1 -> Logical Operator8/2
  Relational Operator18/1 -> Logical Operator8/1
  Logical Operator8/1 -> Switch13/2
  Type20/1 -> Relational Operator23/2
  Type21/1 -> Relational Operator25/2
  Relational Operator25/1 -> Logical Operator9/2
  Relational Operator23/1 -> Logical Operator9/1
  Logical Operator9/1 -> Switch15/2
  Type23/1 -> Relational Operator22/2
  Type22/1 -> Relational Operator26/2
  Relational Operator26/1 -> Logical Operator10/2
  Relational Operator22/1 -> Logical Operator10/1
  Logical Operator10/1 -> Switch14/2
  Type25/1 -> Relational Operator28/2
  Type26/1 -> Relational Operator29/2
  Relational Operator29/1 -> Logical Operator12/2
  Relational Operator28/1 -> Logical Operator12/1
  Logical Operator12/1 -> Switch24/2
  Type40/1 -> Relational Operator27/2
  Type27/1 -> Relational Operator30/2
  Relational Operator30/1 -> Logical Operator13/2
  Relational Operator27/1 -> Logical Operator13/1
  Logical Operator13/1 -> Switch17/2
  Type28/1 -> Relational Operator32/2
  Type29/1 -> Relational Operator33/2
  Relational Operator33/1 -> Logical Operator14/2
  Relational Operator32/1 -> Logical Operator14/1
  Logical Operator14/1 -> Switch19/2
  Type31/1 -> Relational Operator31/2
  Type30/1 -> Relational Operator34/2
  Relational Operator34/1 -> Logical Operator15/2
  Relational Operator31/1 -> Logical Operator15/1
  Logical Operator15/1 -> Switch18/2
  Type32/1 -> Relational Operator36/2
  Type33/1 -> Relational Operator37/2
  Relational Operator37/1 -> Logical Operator16/2
  Relational Operator36/1 -> Logical Operator16/1
  Logical Operator16/1 -> Switch23/2
  Type39/1 -> Relational Operator35/2
  Type34/1 -> Relational Operator38/2
  Relational Operator38/1 -> Logical Operator17/2
  Relational Operator35/1 -> Logical Operator17/1
  Logical Operator17/1 -> Switch20/2
  Type35/1 -> Relational Operator40/2
  Relational Operator40/1 -> Logical Operator18/1
  Logical Operator18/1 -> Switch22/2
  Power3/1 -> Switch9/1
  Power4/1 -> Switch10/1
  Power5/1 -> Switch12/1
  Power6/1 -> Switch11/1
  Power7/1 -> Switch16/1
  Power8/1 -> Switch13/1
  Power9/1 -> Switch15/1
  Power10/1 -> Switch14/1
  Power11/1 -> Switch24/1
  Power12/1 -> Switch17/1
  Power13/1 -> Switch19/1
  Power14/1 -> Switch18/1
  Power15/1 -> Switch23/1
  Power16/1 -> Switch20/1
  Power17/1 -> Switch22/1
  Switch8/1 -> Add2/2
  Switch9/1 -> Add2/3
  Switch12/1 -> Add2/5
  Switch10/1 -> Add2/4
  Switch11/1 -> Add3/1
  Switch16/1 -> Add3/2
  Switch13/1 -> Add3/3
  Switch15/1 -> Add3/4
  Switch14/1 -> Add3/5
  Switch24/1 -> Add4/1
  Switch17/1 -> Add4/2
  Switch19/1 -> Add4/3
  Switch18/1 -> Add4/4
  Switch23/1 -> Add4/5
  Switch20/1 -> Add5/1
  Switch22/1 -> Add5/2
  Switch21/1 -> Add5/3
  Add2/1 -> Add7/1
  Add3/1 -> Add7/2
  Add4/1 -> Add7/3
  Add5/1 -> Add7/4
  Add6/1 -> Add7/5
  Default/1 -> Relational Operator103/2
  Relational Operator103/1 -> Enabled Subsystem1/1(active pulse1)
  WD_OnOff/1 -> Relational Operator103/1, Relational Operator55/2
  Enabled Subsystem1/1(Radiation) -> Add8/2
  Relational Operator55/1 -> Switch29/2
  radiation/1 -> Relational Operator55/1
  Add7/1 -> Switch29/1
  Switch29/1 -> Add8/1
  Integrator3/1 -> PlotResults5/1, Bus Creator4/2  "kw-hr"
  Watts-->kW/1 -> Integrator3/1, Rates/1(Powe_cons), To File1/1, Bus Creator4/3, PlotResults5/2
  Rates/1(Rate) -> Integrator/1
  Integrator/1 -> PlotResults3/1, Bus Creator4/1
  Bus Creator4/1 -> To File5/1
  Rate_season2/1 -> Rates/2(Rate_season2)
  Add8/1 -> PlotResults2/1, Watts-->kW/1

== system Energy_Cost/Air Conditioner/Cost_AA ==
  Powe_cons : Inport
  Rate_season2 : Inport  Port=2
  AcHt : Gain  SaturateOnIntegerOverflow=on  OutDataTypeStr=Inherit: Same as input  ParamDataTypeStr=Inherit: Same as input
  Bus Creator2 : BusCreator  Inputs=3
  Integrator : Integrator
  Integrator3 : Integrator
  PlotResults1 : Scope
  PlotResults2 : Scope
  PlotResults4 : Scope
  Rates : Subsystem
  To File : ToFile  Filename=Pow_Cost_AC  MatrixName=Pow_Cost_AC
  Watts-->kW : Gain  Gain=-1/(3600*1000)  SaturateOnIntegerOverflow=on  OutDataTypeStr=Inherit: Same as input  ParamDataTypeStr=Inherit: Same as input
  Power : Outport  InitialOutput=0
  wires:
  Rates/1(Rate) -> Integrator/1
  Integrator3/1 -> Bus Creator2/2  "kw_hr"
  Bus Creator2/1 -> To File/1, PlotResults1/1
  Integrator/1 -> PlotResults2/1, Bus Creator2/3  "Cost_hr"
  Watts-->kW/1 -> Rates/1(Powe_cons), Integrator3/1, Bus Creator2/1, PlotResults4/1, Power/1
  AcHt/1 -> Watts-->kW/1
  Powe_cons/1 -> AcHt/1
  Rate_season2/1 -> Rates/2(Rate_season2)
